simulink model "q_qube2_bal_lqr"  (R2020b)
settings: Solver=ode1  StartTime=0.0  StopTime=10  FixedStep=0.002  RelTol=1e-3  EnableMultiTasking=on
values from neighbouring files (symbols this model uses):
  K = dlqr(sysd.A,sysd.B,Q1,R1)    [MatrixQandR.m]
undefined symbols (not defined in the file or in its folder): HIL, qc_get_step_size
libraries: simulink_extras x3, quarc_library x3, simulink x1
settings Model: SimulationMode=external  ExtModeTrigDuration=5000000  Creator=MLevis  LastModifiedBy=marco
settings SolverCC: PositivePriorityOrder=on
settings DataIOCC: LimitDataPoints=on  SaveFormat=Array  SignalLoggingSaveFormat=ModelDataLogs  ReturnWorkspaceOutputs=off
settings OptimizationCC: BooleanDataType=off  OptimizeBlockIOStorage=off  BufferReuse=off  GlobalBufferReuse=off  ExpressionFolding=off  ExpressionDepthLimit=2147483647  LocalBlockOutputs=off  InitFltsAndDblsToZero=on  LifeSpan=inf  OptimizeDataStoreBuffers=off  BusAssignmentInplaceUpdate=off
settings DebuggingCC: SaveWithParameterizedLinksMsg=none  UnderspecifiedInitializationDetection=Classic  MergeDetectMultiDrivingBlocksExec=none  SignalResolutionControl=TryResolveAllWithWarning  MultiTaskDSMMsg=warning  MultiTaskCondExecSysMsg=none  FcnCallInpInsideContextMsg=warning  StateNameClashWarn=warning  SFUnexpectedBacktrackingDiag=warning  SFNoUnconditionalDefaultTransitionDiag=warning  SFExecutionAtInitializationDiag=none  ArithmeticOperatorsInVariantConditions=warning
settings HardwareCC: ProdBitPerPointer=32  ProdBitPerSizeT=32  ProdBitPerPtrDiffT=32  ProdLargestAtomicFloat=None  ProdIntDivRoundTo=Undefined  ProdEndianess=Unspecified  ProdWordSize=32  ProdHWDeviceType=32-bit Generic  TargetHWDeviceType=32-bit Generic
settings ModelReferenceCC: PropagateSignalLabelsOutOfModel=off
settings SFSimCC: SimUseLocalCustomCode=off  SimParseCustomCode=off  CustomCodeUndefinedFunction=UseInterfaceOnly
settings RTWCC: Description=QUARC Win64 Target  SystemTargetFile=quarc_win64.tlc  TemplateMakefile=quarc_default_tmf  RTWUseLocalCustomCode=off
settings CodeAppCC: StateflowObjectComments=on
settings STFCustomTargetCC: CPPClassGenCompliant=off
settings GRTTargetCC: TargetLangStandard=C89/C90 (ANSI)  ParMdlRefBuildCompliant=off  CompOptLevelCompliant=off  CombineOutputUpdateFcns=off  MatFileLogging=off  CPPClassGenCompliant=off  GRTInterface=on  UseToolchainInfoCompliant=off  ExtMode=on  ExtModeMexFile=quarc_comm
settings ConfigComp: CovMetricSettings=dw  CovSaveCumulativeToWorkspaceVar=on  CovSaveSingleToWorkspaceVar=on  CovExternalEMLEnable=off  CovSFcnEnable=off

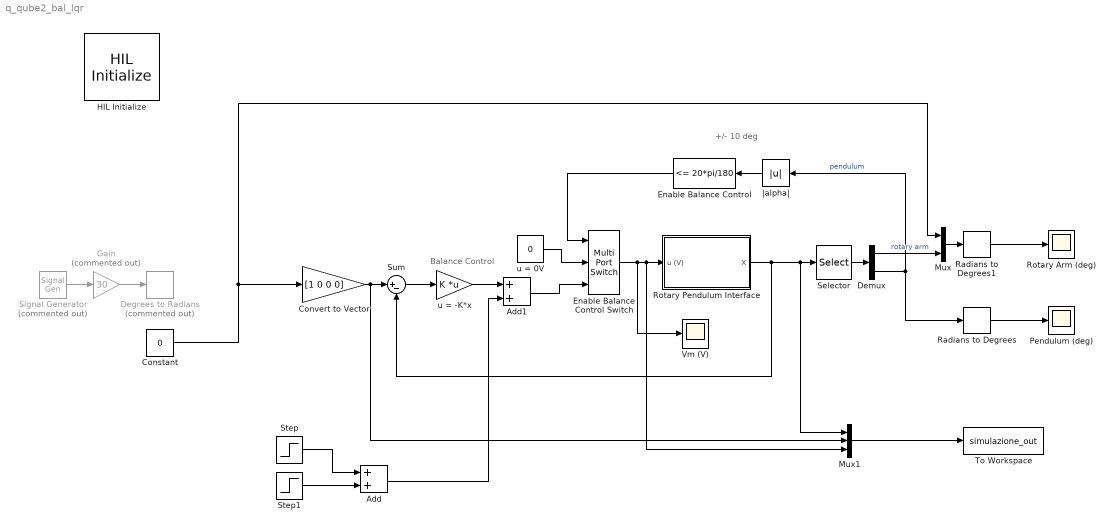
== system q_qube2_bal_lqr ==
  note: +/- 10 deg
  note: Balance Control
  Add : Sum
  Add1 : Sum
  Constant : Constant  Value=0
  Convert to Vector : Gain  Gain=[1 0 0 0]
  Degrees to Radians : simulink_extras/Transformations/Degrees to Radians  Commented=on
  Demux : Demux  Outputs=2
  Enable Balance Control : simulink/Logic and Bit Operations/Compare To Constant  relop=<=  const=20*pi/180  OutDataTypeStr=uint8  ZeroCross=off
  Enable Balance Control Switch : MultiPortSwitch  DataPortOrder=Zero-based contiguous  Inputs=2  zeroidx=on
  Gain : Gain  Commented=on  Gain=30
  HIL Initialize : quarc_library/Data Acquisition/Generic/Configuration/HIL Initialize  object_name=HIL-1  board_type=qube_servo2_usb  board_number=0  board_options=""  exclusive=off  active=off  hardware_clocks=[0]  clock_modes=[]  initial_clock_frequencies=[]  set_clock_params_at_start=off  set_clock_params_at_switch_in=off  set_clock_frequencies_at_start=off  set_clock_frequencies_at_switch_in=off  analog_input_channels=[0]  analog_input_configurations=[]  analog_input_maximums=3  analog_input_minimums=-3  set_analog_input_params_at_start=off  set_analog_input_params_at_switch_in=off  analog_output_channels=[0]  analog_output_maximums=15  analog_output_minimums=-15  initial_analog_outputs=[0]  final_analog_outputs=[0]  watchdog_analog_outputs=0  set_analog_output_params_at_start=off  set_analog_output_params_at_switch_in=off  set_analog_outputs_at_start=on  set_analog_outputs_at_switch_in=off  set_analog_outputs_at_terminate=on  set_analog_outputs_at_switch_out=off  set_analog_outputs_on_watchdog=on  digital_input_channels=[]  digital_output_channels=[0]  digital_output_configuration=[]  initial_digital_outputs=[1]  final_digital_outputs=[0]  watchdog_digital_outputs=[0]  set_digital_output_params_at_start=off  set_digital_output_params_at_switch_in=off  set_digital_outputs_at_start=on  set_digital_outputs_at_switch_in=off  set_digital_outputs_at_terminate=on  set_digital_outputs_at_switch_out=off  set_digital_outputs_on_watchdog=on  encoder_channels=[0:1]  quadrature=[4]  encoder_filter_frequency=[]  initial_encoder_counts=[0]  set_encoder_params_at_start=off  set_encoder_params_at_switch_in=off  set_encoder_counts_at_start=on  set_encoder_counts_at_switch_in=off  pwm_channels=[]  pwm_modes=[]  pwm_frequency=[]  pwm_configuration=[]  pwm_alignment=[]  pwm_polarity=[]  pwm_leading_deadband=[]  pwm_trailing_deadband=[]  initial_pwm_outputs=[]  final_pwm_outputs=[]  watchdog_pwm_outputs=[]  set_pwm_params_at_start=off  set_pwm_params_at_switch_in=off  set_pwm_outputs_at_start=off  set_pwm_outputs_at_switch_in=off  set_pwm_outputs_at_terminate=off  set_pwm_outputs_at_switch_out=off  set_pwm_outputs_on_watchdog=off  other_output_channels=[11000:11002]  initial_other_outputs=[0 1 0]  final_other_outputs=[1 0 0]  watchdog_other_outputs=[0 0 1]  set_other_outputs_at_start=on  set_other_outputs_at_switch_in=off  set_other_outputs_at_terminate=on  set_other_outputs_at_switch_out=off  set_other_outputs_on_watchdog=on
  Mux : Mux  Inputs=2
  Mux1 : Mux  Inputs=3
  Pendulum (deg) : Scope
  Radians to Degrees : simulink_extras/Transformations/Radians to Degrees
  Radians to Degrees1 : simulink_extras/Transformations/Radians to Degrees
  Rotary Arm (deg) : Scope
  Rotary Pendulum Interface : Subsystem
  Selector : Selector  InputPortWidth=4  IndexOptions=Index vector (dialog)  Indices=[1 2]  OutputSizes=1
  Signal Generator : SignalGenerator  Commented=on  WaveForm=square  Frequency=0.125
  Step : Step  Time=5  After=3  SampleTime=0
  Step1 : Step  Time=5.1  Before=3  After=0  SampleTime=0
  Sum : Sum  Inputs=|+-
  To Workspace : ToWorkspace  VariableName=simulazione_out  SaveFormat=Structure With Time  SampleTime=-1
  Vm (V) : Scope
  u = -K*x : Gain  Gain=K  Multiplication=Matrix(K*u)
  u = 0V : Constant  Value=0
  |alpha| : Abs
  wires:
  |alpha|/1 -> Enable Balance Control/1
  Enable Balance Control/1 -> Enable Balance Control Switch/1
  Sum/1 -> u = -K*x/1
  Convert to Vector/1 -> Mux1/2, Sum/1
  Radians to Degrees/1 -> Pendulum (deg)/1
  Radians to Degrees1/1 -> Rotary Arm (deg)/1
  Enable Balance Control Switch/1 -> Vm (V)/1, Mux1/3, Rotary Pendulum Interface/1(u (V))
  u = 0V/1 -> Enable Balance Control Switch/2
  Signal Generator/1 -> Gain/1
  Gain/1 -> Degrees to Radians/1
  Mux/1 -> Radians to Degrees1/1
  Rotary Pendulum Interface/1(X) -> Mux1/1, Selector/1, Sum/2
  Selector/1 -> Demux/1
  Demux/1 -> Mux/2  "rotary arm"
  Demux/2 -> Radians to Degrees/1, |alpha|/1  "pendulum"
  Constant/1 -> Mux/1, Convert to Vector/1
  Mux1/1 -> To Workspace/1
  Step/1 -> Add/1
  Step1/1 -> Add/2
  u = -K*x/1 -> Add1/1
  Add1/1 -> Enable Balance Control Switch/3
  Add/1 -> Add1/2

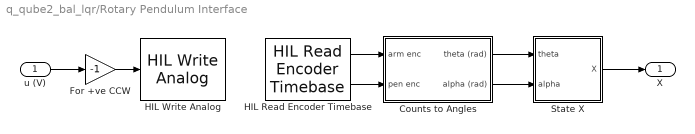
== system q_qube2_bal_lqr/Rotary Pendulum Interface ==
  u (V) : Inport
  Counts to Angles : Subsystem
  For +ve CCW : Gain  Gain=-1
  HIL Read Encoder Timebase : quarc_library/Data Acquisition/Generic/Timebases/HIL Read Encoder Timebase  object_name=HIL-1  clock=0  channels=[0:1]  active=on  vector_output=off  data_type_mode=Inherit via back propagation  data_type=double  overflow_mode=Error on overflow  samples_in_buffer=max(ceil(1/qc_get_step_size), 1)
  HIL Write Analog : quarc_library/Data Acquisition/Generic/Immediate I//O/HIL Write Analog  object_name=HIL-1  channels=0  sample_time=-1  active=off  vector_input=off
  State X : Subsystem
  X : Outport  VectorParamsAs1DForOutWhenUnconnected=off
  wires:
  u (V)/1 -> For +ve CCW/1
  HIL Read Encoder Timebase/2 -> Counts to Angles/2(pen enc)
  For +ve CCW/1 -> HIL Write Analog/1
  HIL Read Encoder Timebase/1 -> Counts to Angles/1(arm enc)
  Counts to Angles/2(alpha (rad)) -> State X/2(alpha)
  Counts to Angles/1(theta (rad)) -> State X/1(theta)
  State X/1(X) -> X/1

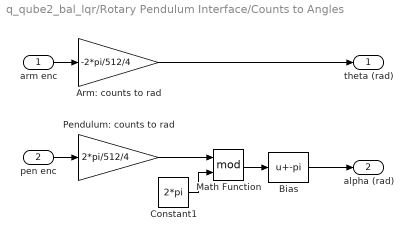
== system q_qube2_bal_lqr/Rotary Pendulum Interface/Counts to Angles ==
  arm enc : Inport
  pen enc : Inport  Port=2
  Arm: counts to rad : Gain  Gain=-2*pi/512/4
  Bias : Bias  Bias=-pi
  Constant1 : Constant  Value=2*pi
  Math Function : Math  Operator=mod  SignedPower=on  SaturateOnIntegerOverflow=on
  Pendulum: counts to rad : Gain  Gain=2*pi/512/4
  theta (rad) : Outport  VectorParamsAs1DForOutWhenUnconnected=off
  alpha (rad) : Outport  Port=2  VectorParamsAs1DForOutWhenUnconnected=off
  wires:
  pen enc/1 -> Pendulum: counts to rad/1
  arm enc/1 -> Arm: counts to rad/1
  Math Function/1 -> Bias/1
  Constant1/1 -> Math Function/2
  Pendulum: counts to rad/1 -> Math Function/1
  Arm: counts to rad/1 -> theta (rad)/1
  Bias/1 -> alpha (rad)/1

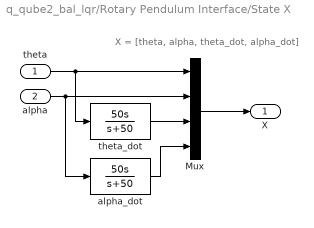
== system q_qube2_bal_lqr/Rotary Pendulum Interface/State X ==
  note: X = [theta, alpha, theta_dot, alpha_dot]
  theta : Inport
  alpha : Inport  Port=2
  Mux : Mux
  alpha_dot : TransferFcn  Numerator=[50 0]  Denominator=[1 50]
  theta_dot : TransferFcn  Numerator=[50 0]  Denominator=[1 50]
  X : Outport  VectorParamsAs1DForOutWhenUnconnected=off
  wires:
  theta_dot/1 -> Mux/3
  alpha_dot/1 -> Mux/4
  alpha/1 -> Mux/2, alpha_dot/1
  Mux/1 -> X/1
  theta/1 -> Mux/1, theta_dot/1
